simulink model "Hydraulika"  (R2013b)
settings: Solver=ode45  StartTime=0.0  StopTime=3  FixedStep=0.001  MaxStep=0.0001  RelTol=1e-5
libraries: simulink x3
settings Model: Creator=Mavitis  LastModifiedBy=Mavitis

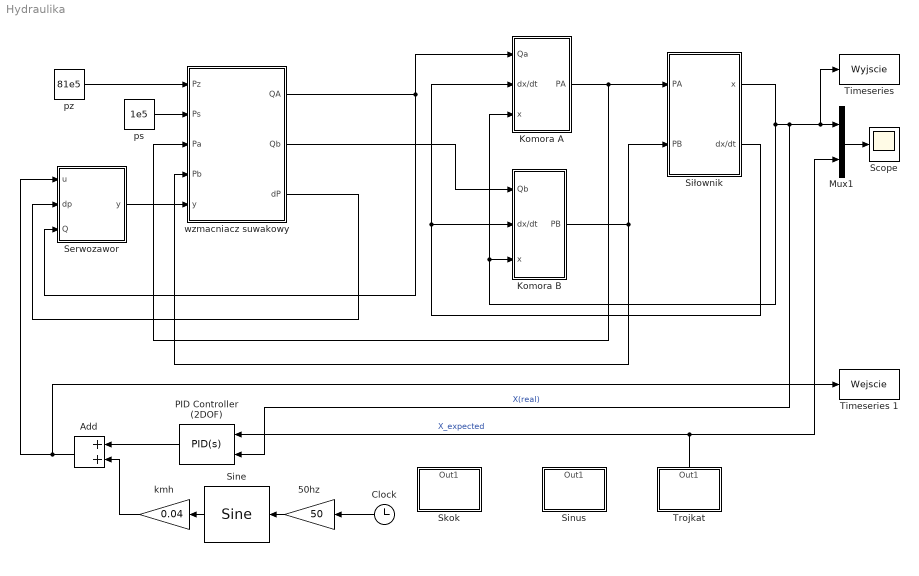
== system Hydraulika ==
  50hz : Gain  Gain=50
  Add : Sum
  Clock : Clock
  Komora A : Subsystem
  Komora B : Subsystem
  Mux1 : Mux  Inputs=2
  PID Controller (2DOF) : simulink/Continuous/PID Controller (2DOF)  Controller=PID  TimeDomain=Continuous-time  SampleTime=1  IntegratorMethod=Forward Euler  FilterMethod=Forward Euler  Form=Parallel  P=180  I=8.18  D=1440  N=0.0125  b=1  c=1  InitialConditionSource=internal  InitialConditionForIntegrator=0  InitialConditionForFilter=0  ExternalReset=none  LimitOutput=off  UpperSaturationLimit=inf  LowerSaturationLimit=-inf  LinearizeAsGain=on  AntiWindupMode=none  Kb=1  TrackingMode=off  Kt=1  PParamMin=[]  PParamMax=[]  IParamMin=[]  IParamMax=[]  DParamMin=[]  DParamMax=[]  NParamMin=[]  NParamMax=[]  bParamMin=[]  bParamMax=[]  cParamMin=[]  cParamMax=[]  KbParamMin=[]  KbParamMax=[]  KtParamMin=[]  KtParamMax=[]  POutMin=[]  POutMax=[]  IOutMin=[]  IOutMax=[]  DOutMin=[]  DOutMax=[]  NOutMin=[]  NOutMax=[]  bOutMin=[]  bOutMax=[]  cOutMin=[]  cOutMax=[]  KbOutMin=[]  KbOutMax=[]  KtOutMin=[]  KtOutMax=[]  IntegratorOutMin=[]  IntegratorOutMax=[]  FilterOutMin=[]  FilterOutMax=[]  SumOutMin=[]  SumOutMax=[]  Sum1OutMin=[]  Sum1OutMax=[]  Sum2OutMin=[]  Sum2OutMax=[]  Sum3OutMin=[]  Sum3OutMax=[]  SumI1OutMin=[]  SumI1OutMax=[]  SumI2OutMin=[]  SumI2OutMax=[]  SumI3OutMin=[]  SumI3OutMax=[]  SumDOutMin=[]  SumDOutMax=[]  SaturationOutMin=[]  SaturationOutMax=[]  IntegratorContinuousStateAttributes=''  IntegratorStateMustResolveToSignalObject=off  IntegratorRTWStateStorageClass=Auto  FilterContinuousStateAttributes=''  FilterStateMustResolveToSignalObject=off  FilterRTWStateStorageClass=Auto
  Scope : Scope
      settings: ShowLegends=on  YMin=0.06875  YMax=0.07425
  Serwozawor : Subsystem
  Sine : simulink/Lookup Tables/Sine  Formula=sin(2*pi*u)  NumDataPoints=(2^5)+1  OutputWordLength=16  InternalRulePriority=Speed
  Sinus : Subsystem
  Siłownik : Subsystem
  Skok : Subsystem
  "Timeseries " : ToWorkspace  VariableName=Wyjscie  SampleTime=-1  SaveFormat=Timeseries
  Timeseries 1 : ToWorkspace  VariableName=Wejscie  SampleTime=-1  SaveFormat=Timeseries
  Trojkat : Subsystem
  kmh : Gain  Gain=0.04
  ps : Constant  Value=1e5
  pz : Constant  Value=81e5
  wzmacniacz suwakowy : Subsystem
  wires:
  PID Controller (2DOF)/1 -> Add/1
  Add/1 -> Timeseries 1/1, Serwozawor/1(u)
  pz/1 -> wzmacniacz suwakowy/1(Pz)
  ps/1 -> wzmacniacz suwakowy/2(Ps)
  wzmacniacz suwakowy/3(dP) -> Serwozawor/2(dp)
  wzmacniacz suwakowy/1(QA) -> Serwozawor/3(Q), Komora A/1(Qa)
  wzmacniacz suwakowy/2(Qb) -> Komora B/1(Qb)
  Sine/1 -> kmh/1
  50hz/1 -> Sine/1
  Clock/1 -> 50hz/1
  Komora A/1("PA ") -> Siłownik/1(PA), wzmacniacz suwakowy/3(Pa)
  Komora B/1("PB ") -> wzmacniacz suwakowy/4(Pb), Siłownik/2(PB)
  Mux1/1 -> Scope/1
  Siłownik/1(x) -> "Timeseries "/1, Mux1/1, PID Controller (2DOF)/2, Komora B/3(x), Komora A/3(x)  "X(real)"
  Siłownik/2(dx/dt) -> Komora B/2(dx/dt), Komora A/2(dx/dt)
  kmh/1 -> Add/2
  Serwozawor/1(y) -> wzmacniacz suwakowy/5(y)
  Trojkat/1(Out1) -> PID Controller (2DOF)/1, Mux1/2  "X_expected"

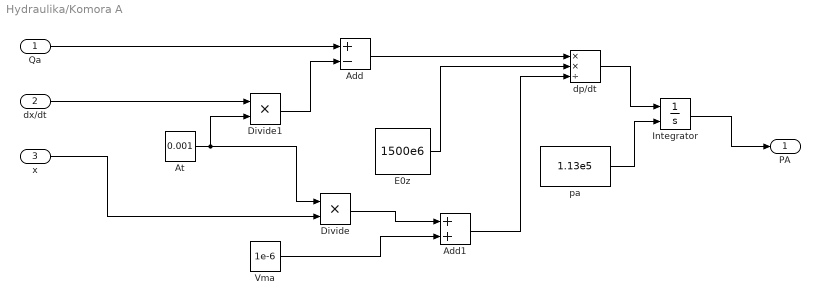
== system Hydraulika/Komora A ==
  Qa : Inport
  dx/dt : Inport  Port=2
  x : Inport  Port=3
  Add : Sum  Inputs=+-
  Add1 : Sum
  At : Constant  Value=0.001
  Divide : Product  Inputs=**
  Divide1 : Product  Inputs=**
  E0z : Constant  Value=1500e6
  Integrator : Integrator  InitialConditionSource=external
  Vma : Constant  Value=1e-6
  dp/dt : Product  Inputs=**/
  pa : Constant  Value=1.13e5
  "PA " : Outport
  wires:
  Qa/1 -> Add/1
  At/1 -> Divide1/2, Divide/1
  dx/dt/1 -> Divide1/1
  Divide1/1 -> Add/2
  E0z/1 -> dp/dt/2
  Add/1 -> dp/dt/1
  x/1 -> Divide/2
  Vma/1 -> Add1/2
  Divide/1 -> Add1/1
  Add1/1 -> dp/dt/3
  dp/dt/1 -> Integrator/1
  Integrator/1 -> "PA "/1
  pa/1 -> Integrator/2

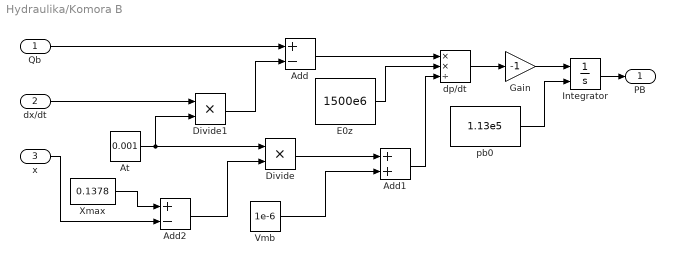
== system Hydraulika/Komora B ==
  Qb : Inport
  dx/dt : Inport  Port=2
  x : Inport  Port=3
  Add : Sum  Inputs=+-
  Add1 : Sum
  Add2 : Sum  Inputs=+-
  At : Constant  Value=0.001
  Divide : Product  Inputs=**
  Divide1 : Product  Inputs=**
  E0z : Constant  Value=1500e6
  Gain : Gain  Gain=-1
  Integrator : Integrator  InitialConditionSource=external
  Vmb : Constant  Value=1e-6
  Xmax : Constant  Value=0.1378
  dp/dt : Product  Inputs=**/
  pb0 : Constant  Value=1.13e5
  "PB " : Outport
  wires:
  Qb/1 -> Add/1
  At/1 -> Divide1/2, Divide/1
  dx/dt/1 -> Divide1/1
  Divide1/1 -> Add/2
  E0z/1 -> dp/dt/2
  Add/1 -> dp/dt/1
  Vmb/1 -> Add1/2
  Divide/1 -> Add1/1
  Add1/1 -> dp/dt/3
  Integrator/1 -> "PB "/1
  x/1 -> Add2/2
  Xmax/1 -> Add2/1
  Add2/1 -> Divide/2
  dp/dt/1 -> Gain/1
  Gain/1 -> Integrator/1
  pb0/1 -> Integrator/2

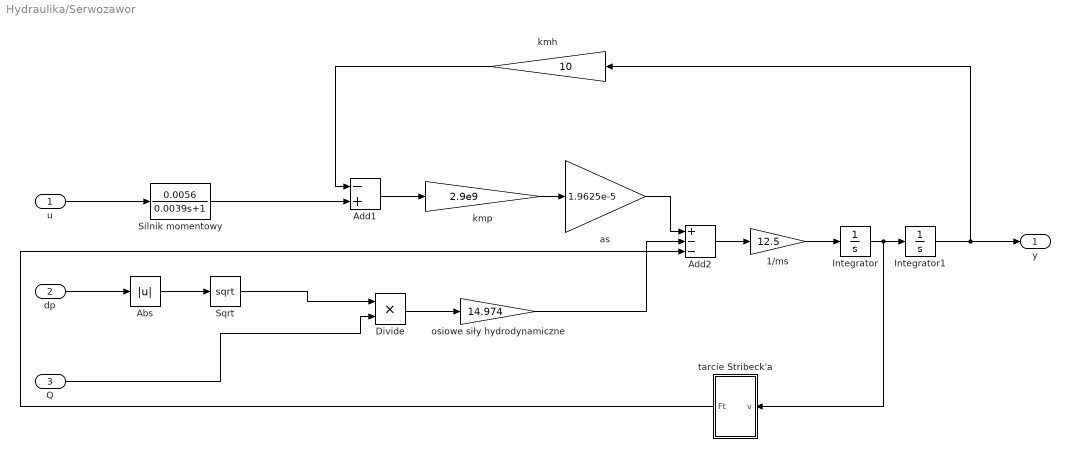
== system Hydraulika/Serwozawor ==
  u : Inport
  dp : Inport  Port=2
  Q : Inport  Port=3
  1/ms : Gain  Gain=12.5
  Abs : Abs
  Add1 : Sum  Inputs=-+
  Add2 : Sum  Inputs=+--
  Divide : Product  Inputs=**
  Integrator : Integrator
  Integrator1 : Integrator
  Silnik momentowy : TransferFcn  Numerator=[0.0056]  Denominator=[0.0039 1]
  Sqrt : Sqrt  SaturateOnIntegerOverflow=on
  as : Gain  Gain=1.9625e-5
  kmh : Gain  Gain=10
  kmp : Gain  Gain=2.9e9
  osiowe siły hydrodynamiczne : Gain  Gain=14.974
  "tarcie Stribeck'a " : Subsystem
  y : Outport
  wires:
  1/ms/1 -> Integrator/1
  osiowe siły hydrodynamiczne/1 -> Add2/2
  Integrator1/1 -> y/1, kmh/1
  Integrator/1 -> "tarcie Stribeck'a "/1(v), Integrator1/1
  kmh/1 -> Add1/1
  kmp/1 -> as/1
  Add1/1 -> kmp/1
  "tarcie Stribeck'a "/1(Ft) -> Add2/3
  as/1 -> Add2/1
  Sqrt/1 -> Divide/1
  Q/1 -> Divide/2
  dp/1 -> Abs/1
  Divide/1 -> osiowe siły hydrodynamiczne/1
  Abs/1 -> Sqrt/1
  Add2/1 -> 1/ms/1
  u/1 -> Silnik momentowy/1
  Silnik momentowy/1 -> Add1/2

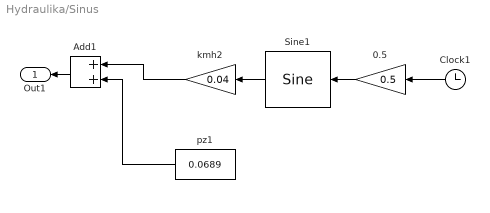
== system Hydraulika/Sinus ==
  0.5 : Gain  Gain=0.5
  Add1 : Sum
  Clock1 : Clock
  Sine1 : simulink/Lookup Tables/Sine  Formula=sin(2*pi*u)  NumDataPoints=(2^5)+1  OutputWordLength=16  InternalRulePriority=Speed
  kmh2 : Gain  Gain=0.04
  pz1 : Constant  Value=0.0689
  Out1 : Outport
  wires:
  Add1/1 -> Out1/1
  Sine1/1 -> kmh2/1
  kmh2/1 -> Add1/1
  pz1/1 -> Add1/2
  0.5/1 -> Sine1/1
  Clock1/1 -> 0.5/1

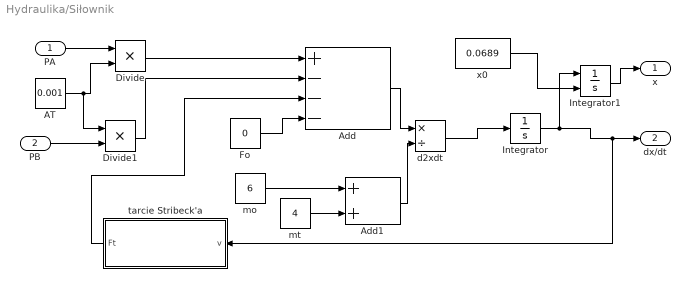
== system Hydraulika/Siłownik ==
  PA : Inport
  PB : Inport  Port=2
  AT : Constant  Value=0.001
  Add : Sum  Inputs=+---
  Add1 : Sum
  Divide : Product  Inputs=**
  Divide1 : Product  Inputs=**
  Fo : Constant  Value=0
  Integrator : Integrator
  Integrator1 : Integrator  InitialConditionSource=external
  d2xdt : Product  Inputs=*/
  "mo " : Constant  Value=6
  mt : Constant  Value=4
  "tarcie Stribeck'a " : Subsystem
  x0 : Constant  Value=0.0689
  x : Outport
  dx/dt : Outport  Port=2
  wires:
  PA/1 -> Divide/1
  AT/1 -> Divide1/1, Divide/2
  PB/1 -> Divide1/2
  Add/1 -> d2xdt/1
  "mo "/1 -> Add1/1
  mt/1 -> Add1/2
  Fo/1 -> Add/4
  "tarcie Stribeck'a "/1(Ft) -> Add/3
  Divide/1 -> Add/1
  Divide1/1 -> Add/2
  Add1/1 -> d2xdt/2
  d2xdt/1 -> Integrator/1
  Integrator/1 -> Integrator1/1, "tarcie Stribeck'a "/1(v), dx/dt/1
  Integrator1/1 -> x/1
  x0/1 -> Integrator1/2

== system Hydraulika/Skok ==
  Add2 : Sum
  Clock2 : Clock
  If : If  IfExpression=u1 < 1.5
  If Action Subsystem : Subsystem  TreatAsAtomicUnit=on
  If Action Subsystem1 : Subsystem  TreatAsAtomicUnit=on
  Out1 : Outport
  wires:
  Clock2/1 -> If/1
  If/1 -> If Action Subsystem/Action
  If/2 -> If Action Subsystem1/Action
  If Action Subsystem/1(Out1) -> Add2/1
  If Action Subsystem1/1(Out1) -> Add2/2
  Add2/1 -> Out1/1

== system Hydraulika/Trojkat ==
  Add2 : Sum
  Clock2 : Clock
  If : If  IfExpression=u1 < 1.5
  If Action Subsystem : Subsystem  TreatAsAtomicUnit=on
  If Action Subsystem1 : Subsystem  TreatAsAtomicUnit=on
  Out1 : Outport
  wires:
  Clock2/1 -> If Action Subsystem1/1(In1), If Action Subsystem/1(In1), If/1
  If/1 -> If Action Subsystem/Action
  If/2 -> If Action Subsystem1/Action
  If Action Subsystem/1(Out1) -> Add2/1
  If Action Subsystem1/1(Out1) -> Add2/2
  Add2/1 -> Out1/1

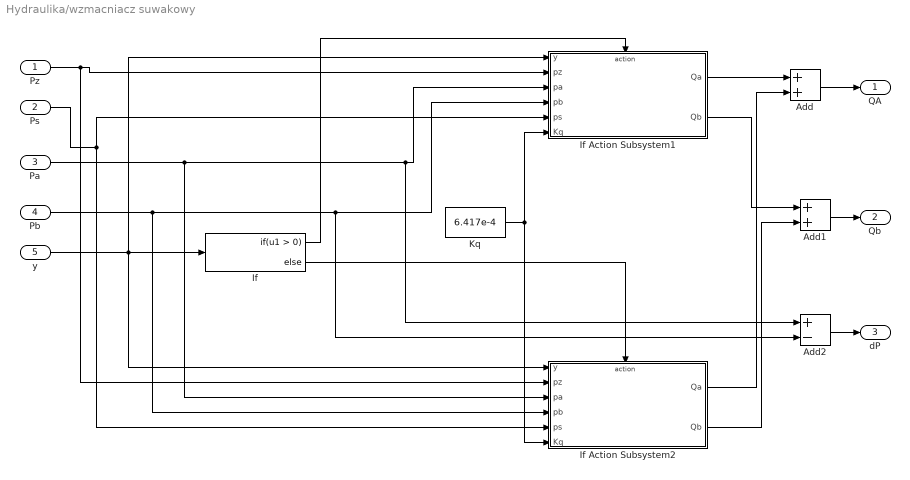
== system Hydraulika/wzmacniacz suwakowy ==
  Pz : Inport
  Ps : Inport  Port=2
  Pa : Inport  Port=3
  Pb : Inport  Port=4
  y : Inport  Port=5
  Add : Sum
  Add1 : Sum
  Add2 : Sum  Inputs=+-
  If : If
  If Action Subsystem1 : Subsystem  TreatAsAtomicUnit=on
  If Action Subsystem2 : Subsystem  TreatAsAtomicUnit=on
  Kq : Constant  Value=6.417e-4
  QA : Outport
  Qb : Outport  Port=2
  dP : Outport  Port=3
  wires:
  y/1 -> If Action Subsystem2/1(y), If Action Subsystem1/1(y), If/1
  If/1 -> If Action Subsystem1/Action
  If/2 -> If Action Subsystem2/Action
  Pz/1 -> If Action Subsystem2/2(pz), If Action Subsystem1/2(pz)
  Pa/1 -> If Action Subsystem2/3(pa), Add2/1, If Action Subsystem1/3(pa)
  Pb/1 -> If Action Subsystem2/4(pb), Add2/2, If Action Subsystem1/4(pb)
  Ps/1 -> If Action Subsystem2/5(ps), If Action Subsystem1/5(ps)
  Kq/1 -> If Action Subsystem2/6(Kq), If Action Subsystem1/6(Kq)
  If Action Subsystem1/1(Qa) -> Add/1
  If Action Subsystem2/1(Qa) -> Add/2
  Add/1 -> QA/1
  If Action Subsystem2/2(Qb) -> Add1/2
  If Action Subsystem1/2(Qb) -> Add1/1
  Add1/1 -> Qb/1
  Add2/1 -> dP/1

== system Hydraulika/Serwozawor/tarcie Stribeck'a  ==
  v : Inport
  Add1 : Sum
  If : If  IfExpression=u1 ~= 0
  If Action Subsystem : Subsystem  TreatAsAtomicUnit=on
  If Action Subsystem1 : Subsystem  TreatAsAtomicUnit=on
  Ft : Outport
  wires:
  Add1/1 -> Ft/1
  If Action Subsystem/1(Out1) -> Add1/1
  If/1 -> If Action Subsystem/Action
  v/1 -> If Action Subsystem1/1(In1), If/1
  If/2 -> If Action Subsystem1/Action
  If Action Subsystem1/1(Out1) -> Add1/2

== system Hydraulika/Siłownik/tarcie Stribeck'a  ==
  v : Inport
  Add1 : Sum
  If : If  IfExpression=u1 ~= 0
  If Action Subsystem : Subsystem  TreatAsAtomicUnit=on
  If Action Subsystem1 : Subsystem  TreatAsAtomicUnit=on
  Ft : Outport
  wires:
  Add1/1 -> Ft/1
  If Action Subsystem/1(Out1) -> Add1/1
  If/1 -> If Action Subsystem/Action
  v/1 -> If Action Subsystem1/1(In1), If/1
  If/2 -> If Action Subsystem1/Action
  If Action Subsystem1/1(Out1) -> Add1/2

== system Hydraulika/Skok/If Action Subsystem ==
  Action Port : ActionPort  ActionType=then
  Add2 : Sum
  x0 : Constant  Value=0.0689
  Out1 : Outport
  wires:
  Add2/1 -> Out1/1
  x0/1 -> Add2/2

== system Hydraulika/Skok/If Action Subsystem1 ==
  Action Port : ActionPort  ActionType=else
  x0 : Constant  Value=0.005
  Out1 : Outport
  wires:
  x0/1 -> Out1/1

== system Hydraulika/Trojkat/If Action Subsystem ==
  In1 : Inport
  Action Port : ActionPort  ActionType=then
  Add2 : Sum
  kmh2 : Gain  Gain=0.02
  x0 : Constant  Value=0.0689
  Out1 : Outport
  wires:
  Add2/1 -> Out1/1
  kmh2/1 -> Add2/1
  In1/1 -> kmh2/1
  x0/1 -> Add2/2

== system Hydraulika/Trojkat/If Action Subsystem1 ==
  In1 : Inport
  Action Port : ActionPort  ActionType=else
  Add2 : Sum
  kmh2 : Gain  Gain=-0.02
  x0 : Constant  Value=0.03
  Out1 : Outport
  wires:
  In1/1 -> kmh2/1
  Add2/1 -> Out1/1
  kmh2/1 -> Add2/1
  x0/1 -> Add2/2

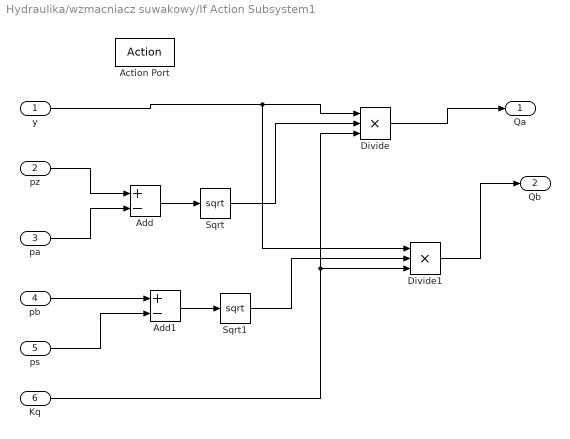
== system Hydraulika/wzmacniacz suwakowy/If Action Subsystem1 ==
  y : Inport
  pz : Inport  Port=2
  pa : Inport  Port=3
  pb : Inport  Port=4
  ps : Inport  Port=5
  Kq : Inport  Port=6
  Action Port : ActionPort  ActionType=then
  Add : Sum  Inputs=+-
  Add1 : Sum  Inputs=+-
  Divide : Product  Inputs=***
  Divide1 : Product  Inputs=***
  Sqrt : Sqrt  SaturateOnIntegerOverflow=on
  Sqrt1 : Sqrt  SaturateOnIntegerOverflow=on
  Qa : Outport
  Qb : Outport  Port=2
  wires:
  Divide/1 -> Qa/1
  Kq/1 -> Divide1/3, Divide/3
  y/1 -> Divide1/1, Divide/1
  pz/1 -> Add/1
  pa/1 -> Add/2
  Add/1 -> Sqrt/1
  Sqrt/1 -> Divide/2
  Add1/1 -> Sqrt1/1
  pb/1 -> Add1/1
  ps/1 -> Add1/2
  Sqrt1/1 -> Divide1/2
  Divide1/1 -> Qb/1

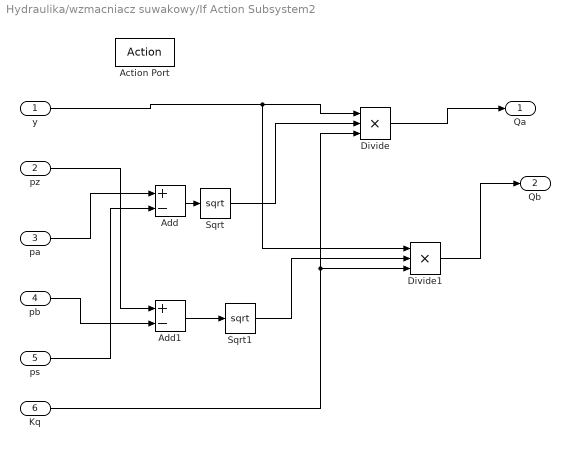
== system Hydraulika/wzmacniacz suwakowy/If Action Subsystem2 ==
  y : Inport
  pz : Inport  Port=2
  pa : Inport  Port=3
  pb : Inport  Port=4
  ps : Inport  Port=5
  Kq : Inport  Port=6
  Action Port : ActionPort  ActionType=else
  Add : Sum  Inputs=+-
  Add1 : Sum  Inputs=+-
  Divide : Product  Inputs=***
  Divide1 : Product  Inputs=***
  Sqrt : Sqrt  SaturateOnIntegerOverflow=on
  Sqrt1 : Sqrt  SaturateOnIntegerOverflow=on
  Qa : Outport
  Qb : Outport  Port=2
  wires:
  Divide/1 -> Qa/1
  Kq/1 -> Divide1/3, Divide/3
  y/1 -> Divide1/1, Divide/1
  Add/1 -> Sqrt/1
  Sqrt/1 -> Divide/2
  Add1/1 -> Sqrt1/1
  Sqrt1/1 -> Divide1/2
  Divide1/1 -> Qb/1
  pa/1 -> Add/1
  ps/1 -> Add/2
  pz/1 -> Add1/1
  pb/1 -> Add1/2

== system Hydraulika/Serwozawor/tarcie Stribeck'a /If Action Subsystem ==
  Action Port : ActionPort  ActionType=then
  Fss : Product  Inputs=***
  g : Constant  Value=9.81
  ms : Constant  Value=0.08
  uss : Constant  Value=0.08
  Out1 : Outport
  wires:
  ms/1 -> Fss/1
  g/1 -> Fss/2
  uss/1 -> Fss/3
  Fss/1 -> Out1/1

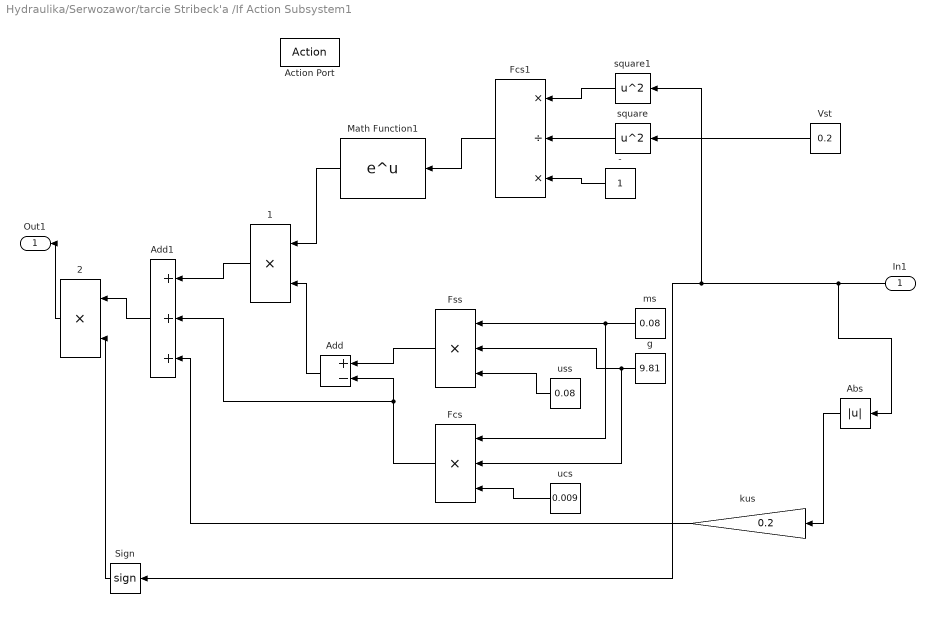
== system Hydraulika/Serwozawor/tarcie Stribeck'a /If Action Subsystem1 ==
  In1 : Inport
  Action Port : ActionPort  ActionType=else
  - : Constant
  1 : Product  Inputs=**
  2 : Product  Inputs=**
  Abs : Abs
  Add : Sum  Inputs=+-
  Add1 : Sum  Inputs=+++
  Fcs : Product  Inputs=***
  Fcs1 : Product  Inputs=*/*
  Fss : Product  Inputs=***
  Math Function1 : Math  SaturateOnIntegerOverflow=on
  Sign : Signum
  Vst : Constant  Value=0.2
  g : Constant  Value=9.81
  kus : Gain  Gain=0.2
  ms : Constant  Value=0.08
  square : Math  Operator=square  SaturateOnIntegerOverflow=on
  square1 : Math  Operator=square  SaturateOnIntegerOverflow=on
  ucs : Constant  Value=0.009
  uss : Constant  Value=0.08
  Out1 : Outport
  wires:
  ms/1 -> Fcs/1, Fss/1
  g/1 -> Fcs/2, Fss/2
  uss/1 -> Fss/3
  -/1 -> Fcs1/3
  square1/1 -> Fcs1/1
  square/1 -> Fcs1/2
  Vst/1 -> square/1
  In1/1 -> Abs/1, Sign/1, square1/1
  Fcs1/1 -> Math Function1/1
  Fss/1 -> Add/1
  Fcs/1 -> Add1/2, Add/2
  Math Function1/1 -> 1/1
  Add/1 -> 1/2
  Abs/1 -> kus/1
  1/1 -> Add1/1
  kus/1 -> Add1/3
  Sign/1 -> 2/2
  Add1/1 -> 2/1
  2/1 -> Out1/1
  ucs/1 -> Fcs/3

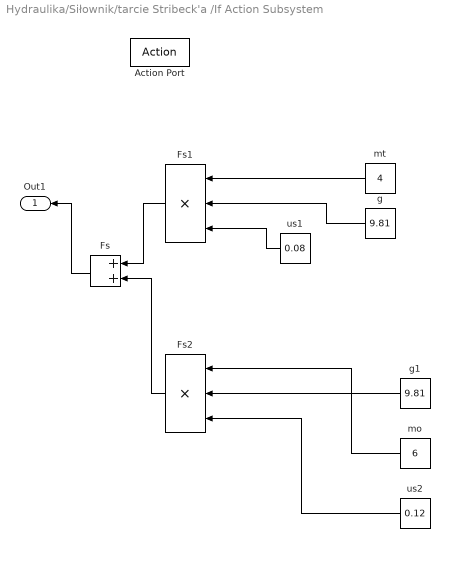
== system Hydraulika/Siłownik/tarcie Stribeck'a /If Action Subsystem ==
  Action Port : ActionPort  ActionType=then
  Fs : Sum
  Fs1 : Product  Inputs=***
  Fs2 : Product  Inputs=***
  g : Constant  Value=9.81
  g1 : Constant  Value=9.81
  mo : Constant  Value=6
  mt : Constant  Value=4
  us1 : Constant  Value=0.08
  us2 : Constant  Value=0.12
  Out1 : Outport
  wires:
  mt/1 -> Fs1/1
  g/1 -> Fs1/2
  us1/1 -> Fs1/3
  mo/1 -> Fs2/1
  g1/1 -> Fs2/2
  us2/1 -> Fs2/3
  Fs2/1 -> Fs/2
  Fs1/1 -> Fs/1
  Fs/1 -> Out1/1

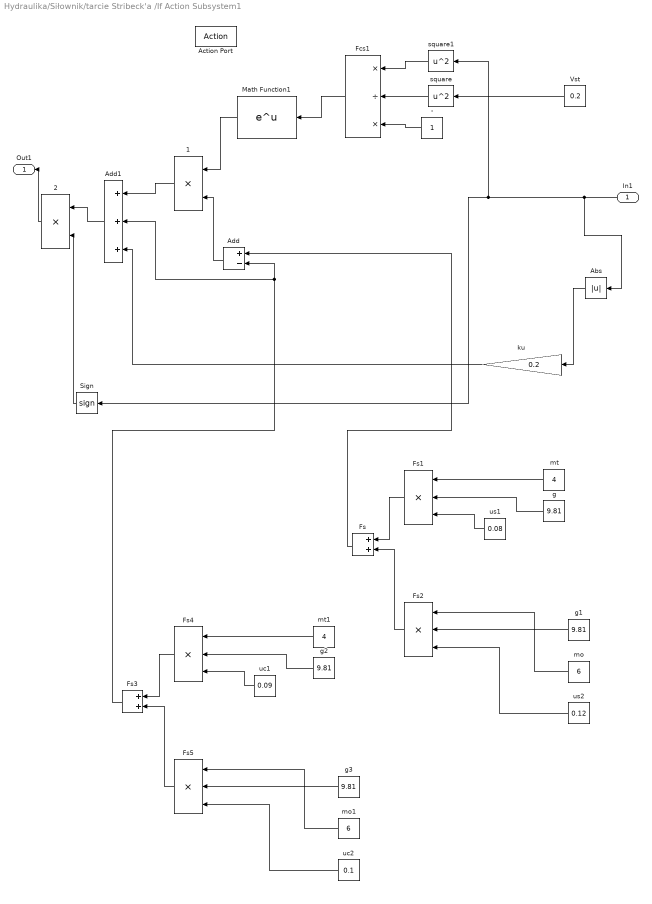
== system Hydraulika/Siłownik/tarcie Stribeck'a /If Action Subsystem1 ==
  In1 : Inport
  Action Port : ActionPort  ActionType=else
  - : Constant
  1 : Product  Inputs=**
  2 : Product  Inputs=**
  Abs : Abs
  Add : Sum  Inputs=+-
  Add1 : Sum  Inputs=+++
  Fcs1 : Product  Inputs=*/*
  Fs : Sum
  Fs{1..2,4..5} (4 alike) : Product  Inputs=***
  Fs3 : Sum
  Math Function1 : Math  SaturateOnIntegerOverflow=on
  Sign : Signum
  Vst : Constant  Value=0.2
  g{,1..3} (4 alike) : Constant  Value=9.81
  ku : Gain  Gain=0.2
  mo : Constant  Value=6
  mo1 : Constant  Value=6
  mt : Constant  Value=4
  mt1 : Constant  Value=4
  square : Math  Operator=square  SaturateOnIntegerOverflow=on
  square1 : Math  Operator=square  SaturateOnIntegerOverflow=on
  uc1 : Constant  Value=0.09
  uc2 : Constant  Value=0.1
  us1 : Constant  Value=0.08
  us2 : Constant  Value=0.12
  Out1 : Outport
  wires:
  -/1 -> Fcs1/3
  square1/1 -> Fcs1/1
  square/1 -> Fcs1/2
  Vst/1 -> square/1
  In1/1 -> Abs/1, Sign/1, square1/1
  Fcs1/1 -> Math Function1/1
  Fs3/1 -> Add1/2, Add/2
  Math Function1/1 -> 1/1
  Add/1 -> 1/2
  Abs/1 -> ku/1
  1/1 -> Add1/1
  ku/1 -> Add1/3
  Sign/1 -> 2/2
  Add1/1 -> 2/1
  2/1 -> Out1/1
  mt/1 -> Fs1/1
  g/1 -> Fs1/2
  us1/1 -> Fs1/3
  mo/1 -> Fs2/1
  g1/1 -> Fs2/2
  us2/1 -> Fs2/3
  Fs2/1 -> Fs/2
  Fs1/1 -> Fs/1
  Fs/1 -> Add/1
  mt1/1 -> Fs4/1
  g2/1 -> Fs4/2
  uc1/1 -> Fs4/3
  mo1/1 -> Fs5/1
  g3/1 -> Fs5/2
  uc2/1 -> Fs5/3
  Fs5/1 -> Fs3/2
  Fs4/1 -> Fs3/1
